simulink model "sfcndemo_stspace"  (R2024a)
settings: Solver=FixedStepDiscrete  StartTime=0.0  StopTime=10.0  FixedStep=1e-3  RelTol=1e-3  EnableMultiTasking=on
Description:
  | Continuous-Time State-Space C-MEX S-function
settings Model: Creator=The MathWorks, Inc.  LastModifiedBy=deshazere
settings SolverCC: AlgebraicLoopSolver=TrustRegion
settings DataIOCC: SaveFormat=Array
settings OptimizationCC: BlockReduction=off  BooleanDataType=off  ExpressionDepthLimit=2147483647  InitFltsAndDblsToZero=on  LifeSpan=inf
settings DebuggingCC: SaveWithParameterizedLinksMsg=none  SignalResolutionControl=TryResolveAllWithWarning  MultiTaskDSMMsg=warning  MultiTaskCondExecSysMsg=none  FcnCallInpInsideContextMsg=warning  UnconnectedInputMsg=warning  UnconnectedOutputMsg=warning  UnconnectedLineMsg=warning  StateNameClashWarn=warning  SFUnexpectedBacktrackingDiag=warning  SFNoUnconditionalDefaultTransitionDiag=warning  SFExecutionAtInitializationDiag=none  ArithmeticOperatorsInVariantConditions=warning
settings HardwareCC: ProdBitPerPointer=32  ProdBitPerSizeT=32  ProdBitPerPtrDiffT=32  ProdLargestAtomicFloat=None  ProdIntDivRoundTo=Undefined  ProdEndianess=Unspecified  ProdWordSize=32  ProdHWDeviceType=32-bit Generic  TargetUnknown=on
settings ModelReferenceCC: EnableRefExpFcnMdlSchedulingChecks=on  PropagateSignalLabelsOutOfModel=off
settings SFSimCC: SimUseLocalCustomCode=off  CustomCodeUndefinedFunction=UseInterfaceOnly
settings RTWCC: RTWUseLocalCustomCode=off  GPUComputeCapability=3.5
settings CodeAppCC: StateflowObjectComments=on
settings GRTTargetCC: TargetFcnLib=ansi_tfl_tmw.mat  TargetLangStandard=C89/C90 (ANSI)  CombineOutputUpdateFcns=off  GRTInterface=on
settings ConfigComp: CovMetricSettings=dw  CovSaveCumulativeToWorkspaceVar=on  CovSaveSingleToWorkspaceVar=on  CovExternalEMLEnable=off

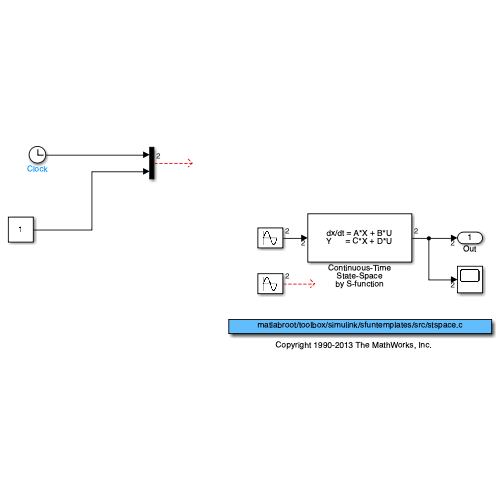
[thumbnail: Simulink's stored preview of the top-level diagram]
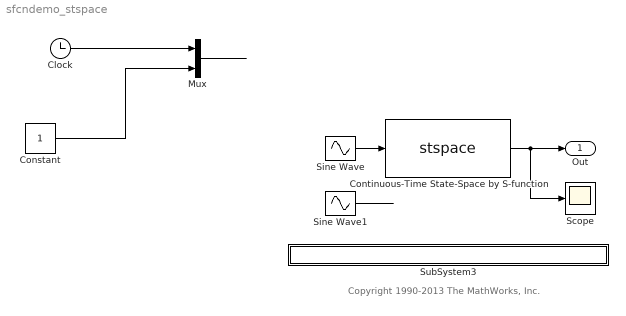
== system sfcndemo_stspace ==
  note: Copyright 1990-2013 The MathWorks, Inc.
  Clock : Clock
  Constant : Constant
  Continuous-Time State-Space by S-function : S-Function  FunctionName=stspace  Parameters=a,b,c,d,x0  SFunctionDeploymentMode=off  EnableBusSupport=off  mask(S-function: stspace){a=[-0.09 -0.01; 1 0], b=[1 -7; 0 -2], c=[0 2; 1 -5], d=[-3 0; 1 0], x0=[]}
      mask prompts: x0 "Initial condition:"
      mask help: This is a S-function block which is the state-space system with dynamic inputs, outputs and states.
      mask Display: disp('dx/dt = A*X + B*U\n Y      = C*X + D*U ');
  Mux : Mux  Inputs=2
  Scope : Scope
  Sine Wave : Sin  Amplitude=[1 2]  SampleTime=0
  Sine Wave1 : Sin  Amplitude=[1 2]  SampleTime=0
  SubSystem3 : Subsystem  mask{filename=stspace.c}
      mask init:
      | x=sfundemo_maskdisp;
      settings: AttributesFormatString=\n  OpenFcn=sfundemo_openfcn
      mask Display: disp(x);
  Out : Outport  InitialOutput=0  VectorParamsAs1DForOutWhenUnconnected=off
  wires:
  Sine Wave/1 -> Continuous-Time State-Space by S-function/1
  Continuous-Time State-Space by S-function/1 -> Out/1, Scope/1
  Sine Wave1/1 -> ?
  Constant/1 -> Mux/2
  Clock/1 -> Mux/1
  Mux/1 -> ?

== system sfcndemo_stspace/SubSystem3 ==
